simulink model "proiect_SCPC_Tamas_Bogdan"  (R2017a)
settings: Solver=ode45  StartTime=0.0  StopTime=1000  RelTol=1e-3
values from neighbouring files (symbols this model uses):
  k = 0.035    [proiect_SCPC_TB.m]    (also in proiect_SCPC_Tamas_Bogdan.m)
  k11 = k2^2 + 4*(k-k3)*k1    (= 0.09336884)    [proiect_SCPC_TB.m]    (also in proiect_SCPC_Tamas_Bogdan.m)
  k12 = 8*(k-k3)    (= 0.2848)    [proiect_SCPC_TB.m]    (also in proiect_SCPC_Tamas_Bogdan.m)
  k13 = 2*(k - k3)    (= 0.0712)    [proiect_SCPC_TB.m]    (also in proiect_SCPC_Tamas_Bogdan.m)
  k2 = -0.015    [proiect_SCPC_TB.m]    (also in proiect_SCPC_Tamas_Bogdan.m)
  keta = 8*10^(-5)    (= 8e-05)    [proiect_SCPC_TB.m]    (also in proiect_SCPC_Tamas_Bogdan.m)
settings Model: Creator=MirrorIce-TerraPower  LastModifiedBy=bogdan.tamas
settings OptimizationCC: LifeSpan=inf
settings DebuggingCC: SFExecutionAtInitializationDiag=none

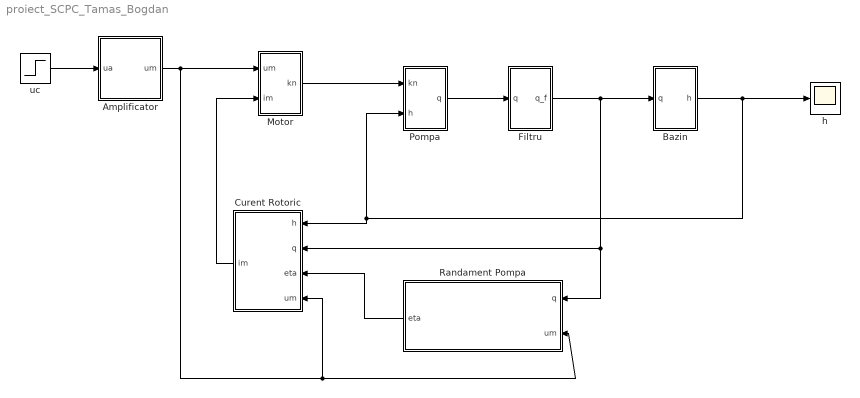
== system proiect_SCPC_Tamas_Bogdan ==
  "Amplificator " : Subsystem
  "Bazin " : Subsystem
  Curent Rotoric : Subsystem
  "Filtru " : Subsystem
  "Motor " : Subsystem
  Pompa : Subsystem
  Randament Pompa : Subsystem
  h : Scope
  "uc " : Step  Time=0  After=5  SampleTime=0
  wires:
  "Amplificator "/1("um ") -> Curent Rotoric/4("um "), Randament Pompa/2("um "), "Motor "/1("um ")
  Curent Rotoric/1("im ") -> "Motor "/2("im ")
  "Motor "/1("kn ") -> Pompa/1(kn)
  Pompa/1("q ") -> "Filtru "/1("q ")
  "Filtru "/1("q_f ") -> "Bazin "/1("q "), Curent Rotoric/2("q "), Randament Pompa/1("q ")
  Randament Pompa/1("eta ") -> Curent Rotoric/3(eta)
  "Bazin "/1(h) -> h/1, Curent Rotoric/1("h "), Pompa/2("h ")
  "uc "/1 -> "Amplificator "/1("ua ")

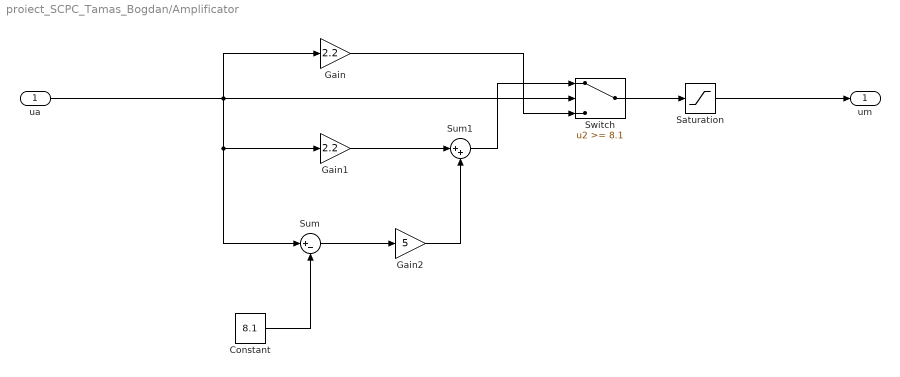
== system proiect_SCPC_Tamas_Bogdan/Amplificator  ==
  "ua " : Inport
  Constant : Constant  Value=8.1
  Gain : Gain  Gain=2.2
  Gain1 : Gain  Gain=2.2
  Gain2 : Gain  Gain=5
  Saturation : Saturate  UpperLimit=22  LowerLimit=0  LinearizeAsGain=off  ZeroCross=off
  Sum : Sum  Inputs=|+-
  Sum1 : Sum  Inputs=|++
  Switch : Switch  Threshold=8.1
  "um " : Outport
  wires:
  "ua "/1 -> Gain1/1, Sum/1, Gain/1, Switch/2
  Saturation/1 -> "um "/1
  Switch/1 -> Saturation/1
  Sum1/1 -> Switch/1
  Gain2/1 -> Sum1/2
  Constant/1 -> Sum/2
  Gain1/1 -> Sum1/1
  Gain/1 -> Switch/3
  Sum/1 -> Gain2/1

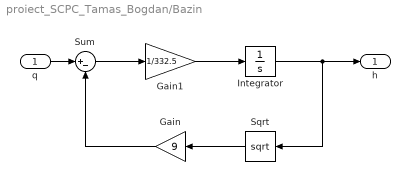
== system proiect_SCPC_Tamas_Bogdan/Bazin  ==
  "q " : Inport
  Gain : Gain  Gain=9
  Gain1 : Gain  Gain=1/332.5
  Integrator : Integrator
  Sqrt : Sqrt  SaturateOnIntegerOverflow=on
  Sum : Sum  Inputs=|+-
  h : Outport
  wires:
  Integrator/1 -> h/1, Sqrt/1
  Sum/1 -> Gain1/1
  Gain/1 -> Sum/2
  "q "/1 -> Sum/1
  Gain1/1 -> Integrator/1
  Sqrt/1 -> Gain/1

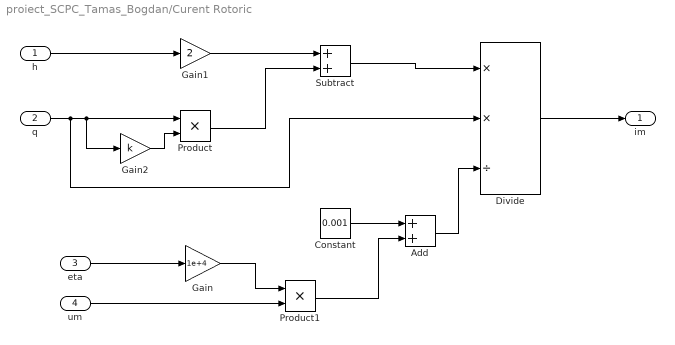
== system proiect_SCPC_Tamas_Bogdan/Curent Rotoric ==
  "h " : Inport
  "q " : Inport  Port=2
  eta : Inport  Port=3
  "um " : Inport  Port=4
  Add : Sum
  Constant : Constant  Value=0.001
  Divide : Product  Inputs=**/
  Gain : Gain  Gain=1e+4
  Gain1 : Gain  Gain=2
  Gain2 : Gain  Gain=k
  Product : Product
  Product1 : Product
  Subtract : Sum
  "im " : Outport
  wires:
  "q "/1 -> Divide/2, Gain2/1, Product/1
  Subtract/1 -> Divide/1
  Product1/1 -> Add/2
  "um "/1 -> Product1/2
  Divide/1 -> "im "/1
  eta/1 -> Gain/1
  Add/1 -> Divide/3
  Product/1 -> Subtract/2
  "h "/1 -> Gain1/1
  Constant/1 -> Add/1
  Gain/1 -> Product1/1
  Gain1/1 -> Subtract/1
  Gain2/1 -> Product/2

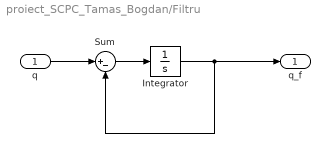
== system proiect_SCPC_Tamas_Bogdan/Filtru  ==
  "q " : Inport
  Integrator : Integrator
  Sum : Sum  Inputs=|+-
  "q_f " : Outport
  wires:
  Integrator/1 -> "q_f "/1, Sum/2
  Sum/1 -> Integrator/1
  "q "/1 -> Sum/1

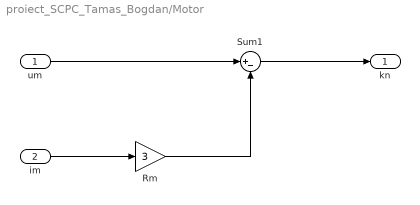
== system proiect_SCPC_Tamas_Bogdan/Motor  ==
  "um " : Inport
  "im " : Inport  Port=2
  Rm : Gain  Gain=3
  Sum1 : Sum  Inputs=|+-
  "kn " : Outport
  wires:
  "um "/1 -> Sum1/1
  "im "/1 -> Rm/1
  Rm/1 -> Sum1/2
  Sum1/1 -> "kn "/1

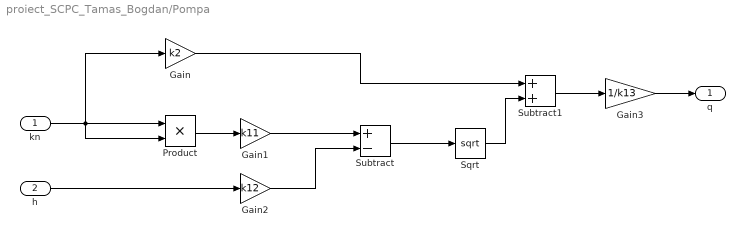
== system proiect_SCPC_Tamas_Bogdan/Pompa ==
  kn : Inport
  "h " : Inport  Port=2
  Gain : Gain  Gain=k2
  Gain1 : Gain  Gain=k11
  Gain2 : Gain  Gain=k12
  Gain3 : Gain  Gain=1/k13
  Product : Product
  Sqrt : Sqrt  SaturateOnIntegerOverflow=on
  Subtract : Sum  Inputs=+-
  Subtract1 : Sum
  "q " : Outport
  wires:
  "h "/1 -> Gain2/1
  Gain1/1 -> Subtract/1
  Subtract/1 -> Sqrt/1
  Subtract1/1 -> Gain3/1
  Gain3/1 -> "q "/1
  Gain2/1 -> Subtract/2
  kn/1 -> Product/2, Product/1, Gain/1
  Product/1 -> Gain1/1
  Sqrt/1 -> Subtract1/2
  Gain/1 -> Subtract1/1

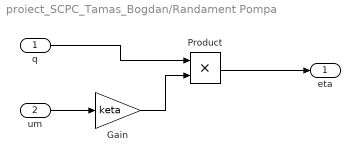
== system proiect_SCPC_Tamas_Bogdan/Randament Pompa ==
  "q " : Inport
  "um " : Inport  Port=2
  Gain : Gain  Gain=keta
  Product : Product
  "eta " : Outport
  wires:
  Product/1 -> "eta "/1
  "um "/1 -> Gain/1
  Gain/1 -> Product/2
  "q "/1 -> Product/1
